simulink model "application_4_si"  (R2017b)
settings: Solver=VariableStepAuto  StartTime=0.0  StopTime=10.0  RelTol=1e-3
libraries: fl_lib x8, nesl_utility x8, elec_lib x5
settings Model: Creator=exybore  LastModifiedBy=exybore

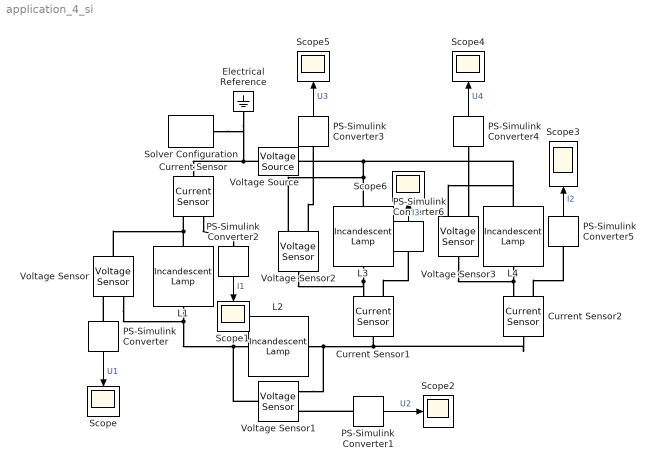
== system application_4_si ==
  Current Sensor : fl_lib/Electrical/Electrical Sensors/Current Sensor
  Current Sensor1 : fl_lib/Electrical/Electrical Sensors/Current Sensor
  Current Sensor2 : fl_lib/Electrical/Electrical Sensors/Current Sensor
  Electrical Reference : fl_lib/Electrical/Electrical Elements/Electrical Reference
  L1 : elec_lib/Passive Devices/Incandescent Lamp  R_param=1  R0=0.000000001 Ohm  R1=0.00000001 Ohm  i0=7 A  i1=6 A  Vrated=12 V  alpha=0.004 1/K  tc=25 ms  initial_state=1  t_fault=inf s  R_fault=1e6 Ohm
      settings: SourceProductName=Simscape Electronics  SourceProductBaseCode=SN
  L2 : elec_lib/Passive Devices/Incandescent Lamp  R_param=1  R0=0.000000001 Ohm  R1=0.00000001 Ohm  i0=0.000000001 A  i1=0.00000001 A  Vrated=12 V  alpha=0.004 1/K  tc=25 ms  initial_state=1  t_fault=inf s  R_fault=1e6 Ohm
      settings: SourceProductName=Simscape Electronics  SourceProductBaseCode=SN
  L3 : elec_lib/Passive Devices/Incandescent Lamp  R_param=1  R0=0.000000001 Ohm  R1=0.00000001 Ohm  i0=0.000000001 A  i1=0.00000001 A  Vrated=12 V  alpha=0.004 1/K  tc=25 ms  initial_state=1  t_fault=inf s  R_fault=1e6 Ohm
      settings: SourceProductName=Simscape Electronics  SourceProductBaseCode=SN
  L4 : elec_lib/Passive Devices/Incandescent Lamp  R_param=1  R0=0.00000001 Ohm  R1=0.0000001 Ohm  i0=70 A  i1=10 A  Vrated=12 V  alpha=0.004 1/K  tc=25 ms  initial_state=1  t_fault=inf s  R_fault=1e6 Ohm
      settings: SourceProductName=Simscape Electronics  SourceProductBaseCode=SN
  PS-Simulink Converter{,1..6} (7 alike) : nesl_utility/PS-Simulink Converter  PhysicalDomain=network_engine_domain  SubClassName=ps_output  LeftPortType=input  RightPortType=output  PseudoPeriodic=off  Frequencies=[]  Unit=1  AffineConversion=off
  Scope{,1..6} (7 alike) : Scope
  Solver Configuration : nesl_utility/Solver Configuration  PhysicalDomain=network_engine_domain  SubClassName=solver  LeftPortType=input  RightPortType=generic  Accelerate=off  Tones=[]  Harmonics=[]  SimulateNoise=off  Profile=off  UseLocalSampling=off  EnableSwitchedLinearOptims=on  FrequencyDomain=off  UseCCode=off  RelTol=0.001  AbsTol=1e-06  MinStep=1e-09  ToWorkspace=off  RevertToSquareIcSolve=off  NumHomotopyIterations=100  PhasorMode=off  PhasorModeNumHarmonics=1  DoDC=off  ResidualTolerance=1e-09  UseLocalSolver=off  LocalSolverChoice=NE_BACKWARD_EULER_ADVANCER  LocalSolverSampleTime=0.001  DoFixedCost=off  MaxNonlinIter=3  MaxModeIter=2  LinearAlgebra=Sparse  DelaysMemoryBudget=1024  AutomaticFiltering=on  FilteringTimeConstant=0.001
  Voltage Sensor{,1..3} (4 alike) : fl_lib/Electrical/Electrical Sensors/Voltage Sensor
  Voltage Source : elec_lib/Sources/Voltage Source  dc_voltage=12 V  ac_voltage=0 V  ac_shift=0 rad  ac_frequency=60 Hz  noise_mode=0  PSD=0 V^2/Hz  repeatability=1  auto_seed=3886434167  user_seed=0  sample_time=1e-3 s  i_specify=off  i_priority=None  i=0 A  i_nominal_specify=off  i_nominal_unit=A  i_nominal_value=1  v_specify=off  v_priority=None  v=0 V  v_nominal_specify=off  v_nominal_unit=V  v_nominal_value=1
      settings: SourceProductName=Simscape Electronics  SourceProductBaseCode=SN
  wires:
  PS-Simulink Converter/1 -> Scope/1  "U1"
  PS-Simulink Converter2/1 -> Scope1/1  "I1"
  PS-Simulink Converter1/1 -> Scope2/1  "U2"
  PS-Simulink Converter5/1 -> Scope3/1  "I2"
  PS-Simulink Converter4/1 -> Scope4/1  "U4"
  PS-Simulink Converter3/1 -> Scope5/1  "U3"
  PS-Simulink Converter6/1 -> Scope6/1  "I3"
  connections:
  L1/LConn1 -- Voltage Sensor/LConn1 -- Current Sensor/RConn2
  Voltage Source/LConn1 -- Solver Configuration/RConn1 -- Electrical Reference/LConn1 -- Current Sensor/LConn1
  L1/RConn1 -- Voltage Sensor/RConn2 -- Voltage Sensor1/LConn1 -- L2/LConn1
  L2/RConn1 -- Voltage Sensor1/RConn2 -- Current Sensor2/LConn1 -- Current Sensor1/LConn1
  L3/LConn1 -- Voltage Sensor2/LConn1 -- Current Sensor1/RConn2
  L4/LConn1 -- Voltage Sensor3/LConn1 -- Current Sensor2/RConn2
  L3/RConn1 -- Voltage Sensor2/RConn2 -- Voltage Sensor3/RConn2 -- L4/RConn1 -- Voltage Source/RConn1
  PS-Simulink Converter/LConn1 -- Voltage Sensor/RConn1
  PS-Simulink Converter1/LConn1 -- Voltage Sensor1/RConn1
  Current Sensor/RConn1 -- PS-Simulink Converter2/LConn1
  Voltage Sensor2/RConn1 -- PS-Simulink Converter3/LConn1
  PS-Simulink Converter4/LConn1 -- Voltage Sensor3/RConn1
  Current Sensor2/RConn1 -- PS-Simulink Converter5/LConn1
  Current Sensor1/RConn1 -- PS-Simulink Converter6/LConn1
